simulink model "PID_nivel_TEMP"  (R2016a)
settings: Solver=VariableStepAuto  StartTime=0.0  StopTime=50  RelTol=1e-3
libraries: simulink x4
settings Model: Creator=Caeta  LastModifiedBy=Caeta

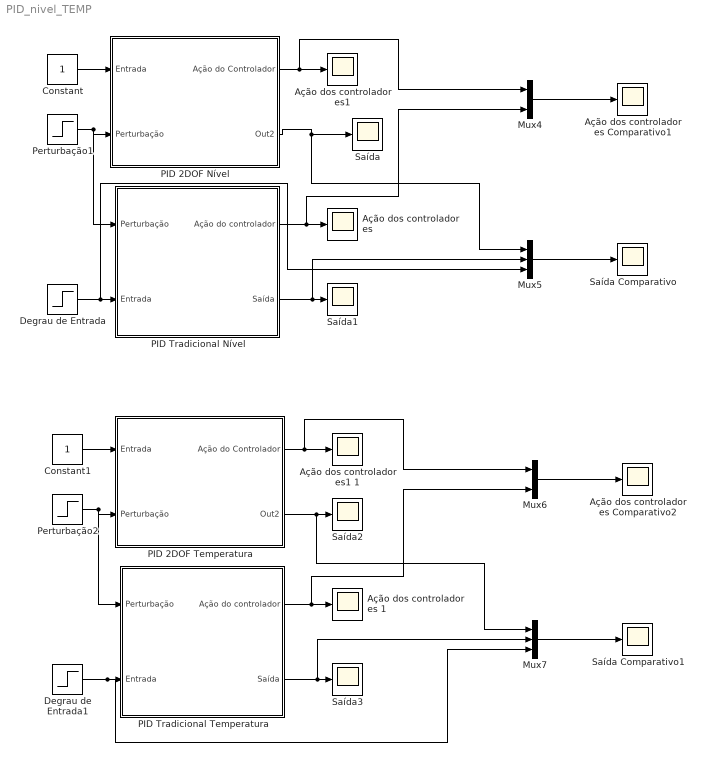
== system PID_nivel_TEMP ==
  "Ação dos controladores " : Scope
  Ação dos controladores 1 : Scope
  Ação dos controladores Comparativo1 : Scope
  Ação dos controladores Comparativo2 : Scope
  "Ação dos controladores1 " : Scope
  Ação dos controladores1 1 : Scope
  Constant : Constant
  Constant1 : Constant
  Degrau de Entrada : Step  SampleTime=0
  Degrau de Entrada1 : Step  Time=0  SampleTime=0
  Mux4 : Mux  Inputs=2
  Mux5 : Mux  Inputs=3
  Mux6 : Mux  Inputs=2
  Mux7 : Mux  Inputs=3
  PID 2DOF Nível : Subsystem
  PID 2DOF Temperatura : Subsystem
  PID Tradicional Nível : Subsystem
  PID Tradicional Temperatura : Subsystem
  Perturbação1 : Step  Time=30  SampleTime=0
  Perturbação2 : Step  Time=30  SampleTime=0
  Saída{,1..3} (4 alike) : Scope
  Saída Comparativo : Scope
  Saída Comparativo1 : Scope
  wires:
  Mux4/1 -> Ação dos controladores Comparativo1/1
  Degrau de Entrada/1 -> Mux5/3, PID Tradicional Nível/2(Entrada)
  PID Tradicional Nível/1(Ação do controlador) -> Mux4/2, "Ação dos controladores "/1
  PID Tradicional Nível/2(Saída) -> Mux5/2, Saída1/1
  Constant/1 -> PID 2DOF Nível/1(Entrada)
  PID 2DOF Nível/2(Out2) -> Mux5/1, Saída/1
  PID 2DOF Nível/1(Ação do Controlador) -> Mux4/1, "Ação dos controladores1 "/1
  Perturbação1/1 -> PID Tradicional Nível/1(Perturbação), PID 2DOF Nível/2(Perturbação)
  Mux5/1 -> Saída Comparativo/1
  Mux6/1 -> Ação dos controladores Comparativo2/1
  Degrau de Entrada1/1 -> Mux7/3, PID Tradicional Temperatura/2(Entrada)
  PID Tradicional Temperatura/1(Ação do controlador) -> Mux6/2, Ação dos controladores 1/1
  PID Tradicional Temperatura/2(Saída) -> Mux7/2, Saída3/1
  Constant1/1 -> PID 2DOF Temperatura/1(Entrada)
  PID 2DOF Temperatura/2(Out2) -> Mux7/1, Saída2/1
  PID 2DOF Temperatura/1(Ação do Controlador) -> Mux6/1, Ação dos controladores1 1/1
  Perturbação2/1 -> PID Tradicional Temperatura/1(Perturbação), PID 2DOF Temperatura/2(Perturbação)
  Mux7/1 -> Saída Comparativo1/1

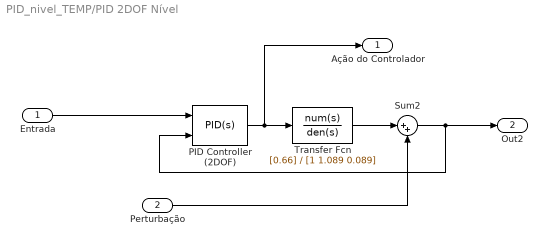
== system PID_nivel_TEMP/PID 2DOF Nível ==
  Entrada : Inport
  Perturbação : Inport  Port=2
  PID Controller (2DOF) : simulink/Continuous/PID Controller (2DOF)  Controller=PID  TimeDomain=Continuous-time  SampleTime=-1  IntegratorMethod=Forward Euler  FilterMethod=Forward Euler  Form=Parallel  UseFilter=on  ControllerParametersSource=internal  P=1.87  I=0.41  D=1.47  N=1  b=0.208  c=0.208  InitialConditionSource=internal  InitialConditionForIntegrator=0  InitialConditionForFilter=0  ExternalReset=none  LimitOutput=off  UpperSaturationLimit=inf  LowerSaturationLimit=-inf  LinearizeAsGain=on  AntiWindupMode=none  Kb=1  TrackingMode=off  Kt=1  PParamMin=[]  PParamMax=[]  IParamMin=[]  IParamMax=[]  DParamMin=[]  DParamMax=[]  NParamMin=[]  NParamMax=[]  bParamMin=[]  bParamMax=[]  cParamMin=[]  cParamMax=[]  KbParamMin=[]  KbParamMax=[]  KtParamMin=[]  KtParamMax=[]  POutMin=[]  POutMax=[]  IOutMin=[]  IOutMax=[]  DOutMin=[]  DOutMax=[]  NOutMin=[]  NOutMax=[]  bOutMin=[]  bOutMax=[]  cOutMin=[]  cOutMax=[]  KbOutMin=[]  KbOutMax=[]  KtOutMin=[]  KtOutMax=[]  IntegratorOutMin=[]  IntegratorOutMax=[]  FilterOutMin=[]  FilterOutMax=[]  SumOutMin=[]  SumOutMax=[]  Sum1OutMin=[]  Sum1OutMax=[]  Sum2OutMin=[]  Sum2OutMax=[]  Sum3OutMin=[]  Sum3OutMax=[]  SumI1OutMin=[]  SumI1OutMax=[]  SumI2OutMin=[]  SumI2OutMax=[]  SumI3OutMin=[]  SumI3OutMax=[]  SumDOutMin=[]  SumDOutMax=[]  SaturationOutMin=[]  SaturationOutMax=[]  IntegratorContinuousStateAttributes=''  IntegratorStateMustResolveToSignalObject=off  IntegratorRTWStateStorageClass=Auto  FilterContinuousStateAttributes=''  FilterStateMustResolveToSignalObject=off  FilterRTWStateStorageClass=Auto  DifferentiatorICPrevScaledInput=0  DifferentiatorOutMin=[]  DifferentiatorOutMax=[]
  Sum2 : Sum  Inputs=|++
  Transfer Fcn : TransferFcn  Numerator=[0.66]  Denominator=[1 1.089 0.089]
  Ação do Controlador : Outport
  Out2 : Outport  Port=2
  wires:
  Sum2/1 -> Out2/1, PID Controller (2DOF)/2
  Perturbação/1 -> Sum2/2
  Entrada/1 -> PID Controller (2DOF)/1
  PID Controller (2DOF)/1 -> Ação do Controlador/1, Transfer Fcn/1
  Transfer Fcn/1 -> Sum2/1

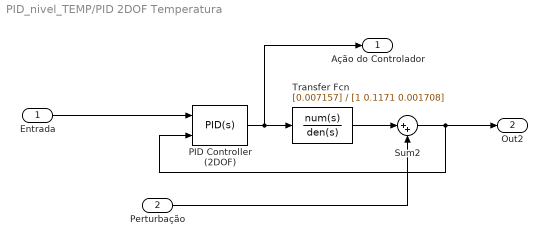
== system PID_nivel_TEMP/PID 2DOF Temperatura ==
  Entrada : Inport
  Perturbação : Inport  Port=2
  PID Controller (2DOF) : simulink/Continuous/PID Controller (2DOF)  Controller=PID  TimeDomain=Continuous-time  SampleTime=-1  IntegratorMethod=Forward Euler  FilterMethod=Forward Euler  Form=Parallel  UseFilter=on  ControllerParametersSource=internal  P=40.8  I=3.02  D=137  N=1  b=0.803  c=0.445  InitialConditionSource=internal  InitialConditionForIntegrator=0  InitialConditionForFilter=0  ExternalReset=none  LimitOutput=off  UpperSaturationLimit=inf  LowerSaturationLimit=-inf  LinearizeAsGain=on  AntiWindupMode=none  Kb=1  TrackingMode=off  Kt=1  PParamMin=[]  PParamMax=[]  IParamMin=[]  IParamMax=[]  DParamMin=[]  DParamMax=[]  NParamMin=[]  NParamMax=[]  bParamMin=[]  bParamMax=[]  cParamMin=[]  cParamMax=[]  KbParamMin=[]  KbParamMax=[]  KtParamMin=[]  KtParamMax=[]  POutMin=[]  POutMax=[]  IOutMin=[]  IOutMax=[]  DOutMin=[]  DOutMax=[]  NOutMin=[]  NOutMax=[]  bOutMin=[]  bOutMax=[]  cOutMin=[]  cOutMax=[]  KbOutMin=[]  KbOutMax=[]  KtOutMin=[]  KtOutMax=[]  IntegratorOutMin=[]  IntegratorOutMax=[]  FilterOutMin=[]  FilterOutMax=[]  SumOutMin=[]  SumOutMax=[]  Sum1OutMin=[]  Sum1OutMax=[]  Sum2OutMin=[]  Sum2OutMax=[]  Sum3OutMin=[]  Sum3OutMax=[]  SumI1OutMin=[]  SumI1OutMax=[]  SumI2OutMin=[]  SumI2OutMax=[]  SumI3OutMin=[]  SumI3OutMax=[]  SumDOutMin=[]  SumDOutMax=[]  SaturationOutMin=[]  SaturationOutMax=[]  IntegratorContinuousStateAttributes=''  IntegratorStateMustResolveToSignalObject=off  IntegratorRTWStateStorageClass=Auto  FilterContinuousStateAttributes=''  FilterStateMustResolveToSignalObject=off  FilterRTWStateStorageClass=Auto  DifferentiatorICPrevScaledInput=0  DifferentiatorOutMin=[]  DifferentiatorOutMax=[]
  Sum2 : Sum  Inputs=|++
  Transfer Fcn : TransferFcn  Numerator=[0.007157]  Denominator=[1 0.1171 0.001708]
  Ação do Controlador : Outport
  Out2 : Outport  Port=2
  wires:
  Sum2/1 -> Out2/1, PID Controller (2DOF)/2
  Perturbação/1 -> Sum2/2
  Entrada/1 -> PID Controller (2DOF)/1
  PID Controller (2DOF)/1 -> Ação do Controlador/1, Transfer Fcn/1
  Transfer Fcn/1 -> Sum2/1

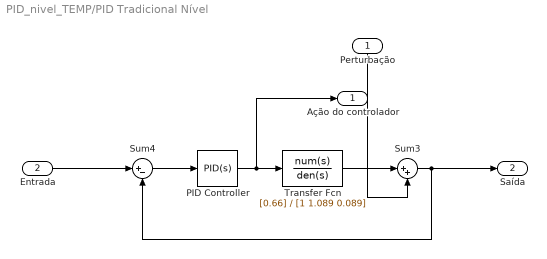
== system PID_nivel_TEMP/PID Tradicional Nível ==
  Perturbação : Inport
  Entrada : Inport  Port=2
  PID Controller : simulink/Continuous/PID Controller  Controller=PID  TimeDomain=Continuous-time  SampleTime=-1  IntegratorMethod=Forward Euler  FilterMethod=Forward Euler  Form=Parallel  UseFilter=on  ControllerParametersSource=internal  P=1.87  I=0.41  D=1.47  N=1  InitialConditionSource=internal  InitialConditionForIntegrator=0  InitialConditionForFilter=0  ExternalReset=none  LimitOutput=off  UpperSaturationLimit=inf  LowerSaturationLimit=-inf  LinearizeAsGain=on  AntiWindupMode=none  Kb=1  TrackingMode=off  Kt=1  PParamMin=[]  PParamMax=[]  IParamMin=[]  IParamMax=[]  DParamMin=[]  DParamMax=[]  NParamMin=[]  NParamMax=[]  KbParamMin=[]  KbParamMax=[]  KtParamMin=[]  KtParamMax=[]  POutMin=[]  POutMax=[]  IOutMin=[]  IOutMax=[]  DOutMin=[]  DOutMax=[]  NOutMin=[]  NOutMax=[]  KbOutMin=[]  KbOutMax=[]  KtOutMin=[]  KtOutMax=[]  IntegratorOutMin=[]  IntegratorOutMax=[]  FilterOutMin=[]  FilterOutMax=[]  SumOutMin=[]  SumOutMax=[]  SumI1OutMin=[]  SumI1OutMax=[]  SumI2OutMin=[]  SumI2OutMax=[]  SumI3OutMin=[]  SumI3OutMax=[]  SumDOutMin=[]  SumDOutMax=[]  SaturationOutMin=[]  SaturationOutMax=[]  IntegratorContinuousStateAttributes=''  IntegratorStateMustResolveToSignalObject=off  IntegratorRTWStateStorageClass=Auto  FilterContinuousStateAttributes=''  FilterStateMustResolveToSignalObject=off  FilterRTWStateStorageClass=Auto  DifferentiatorICPrevScaledInput=0  DifferentiatorOutMin=[]  DifferentiatorOutMax=[]
  Sum3 : Sum  Inputs=|++
  Sum4 : Sum  Inputs=|+-
  Transfer Fcn : TransferFcn  Numerator=[0.66]  Denominator=[1 1.089 0.089]
  Ação do controlador : Outport
  Saída : Outport  Port=2
  wires:
  Perturbação/1 -> Sum3/2
  Sum4/1 -> PID Controller/1
  Sum3/1 -> Saída/1, Sum4/2
  PID Controller/1 -> Transfer Fcn/1, Ação do controlador/1
  Entrada/1 -> Sum4/1
  Transfer Fcn/1 -> Sum3/1

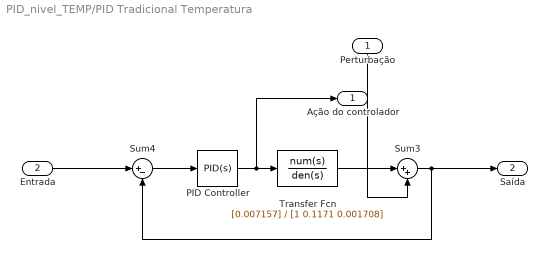
== system PID_nivel_TEMP/PID Tradicional Temperatura ==
  Perturbação : Inport
  Entrada : Inport  Port=2
  PID Controller : simulink/Continuous/PID Controller  Controller=PID  TimeDomain=Continuous-time  SampleTime=-1  IntegratorMethod=Forward Euler  FilterMethod=Forward Euler  Form=Parallel  UseFilter=on  ControllerParametersSource=internal  P=40.8  I=3.02  D=137  N=1  InitialConditionSource=internal  InitialConditionForIntegrator=0  InitialConditionForFilter=0  ExternalReset=none  LimitOutput=off  UpperSaturationLimit=inf  LowerSaturationLimit=-inf  LinearizeAsGain=on  AntiWindupMode=none  Kb=1  TrackingMode=off  Kt=1  PParamMin=[]  PParamMax=[]  IParamMin=[]  IParamMax=[]  DParamMin=[]  DParamMax=[]  NParamMin=[]  NParamMax=[]  KbParamMin=[]  KbParamMax=[]  KtParamMin=[]  KtParamMax=[]  POutMin=[]  POutMax=[]  IOutMin=[]  IOutMax=[]  DOutMin=[]  DOutMax=[]  NOutMin=[]  NOutMax=[]  KbOutMin=[]  KbOutMax=[]  KtOutMin=[]  KtOutMax=[]  IntegratorOutMin=[]  IntegratorOutMax=[]  FilterOutMin=[]  FilterOutMax=[]  SumOutMin=[]  SumOutMax=[]  SumI1OutMin=[]  SumI1OutMax=[]  SumI2OutMin=[]  SumI2OutMax=[]  SumI3OutMin=[]  SumI3OutMax=[]  SumDOutMin=[]  SumDOutMax=[]  SaturationOutMin=[]  SaturationOutMax=[]  IntegratorContinuousStateAttributes=''  IntegratorStateMustResolveToSignalObject=off  IntegratorRTWStateStorageClass=Auto  FilterContinuousStateAttributes=''  FilterStateMustResolveToSignalObject=off  FilterRTWStateStorageClass=Auto  DifferentiatorICPrevScaledInput=0  DifferentiatorOutMin=[]  DifferentiatorOutMax=[]
  Sum3 : Sum  Inputs=|++
  Sum4 : Sum  Inputs=|+-
  Transfer Fcn : TransferFcn  Numerator=[0.007157]  Denominator=[1 0.1171 0.001708]
  Ação do controlador : Outport
  Saída : Outport  Port=2
  wires:
  Transfer Fcn/1 -> Sum3/1
  Perturbação/1 -> Sum3/2
  Sum4/1 -> PID Controller/1
  Sum3/1 -> Saída/1, Sum4/2
  PID Controller/1 -> Transfer Fcn/1, Ação do controlador/1
  Entrada/1 -> Sum4/1
